simulink model "Table_airbus_v2"  (R2021b)
settings: Solver=VariableStepAuto  StartTime=0.0  StopTime=60*1.5  MaxStep=0.1  RelTol=0.01
undefined symbols (not defined in the file): X, Y, Z
libraries: sm_lib x907, fl_lib x68, nesl_utility x53, sdl_lib x10, simulink x7, ee_lib x7, slpidlib x6, simulink_extras x4
(part 4 of 18)

== system Table_airbus_v2/Vérin électrique Levage/Capteur mecanique Z1 ==
  Bus Creator : BusCreator  Inputs=4
  Ideal Rotational Motion Sensor1 : fl_lib/Mechanical/Mechanical Sensors/Ideal Rotational Motion Sensor  wrap_angle=simscape.enum.onoff.off  offset=0 deg
  Ideal Torque Sensor1 : fl_lib/Mechanical/Mechanical Sensors/Ideal Torque Sensor
  Mechanical Rotational Reference6 : fl_lib/Mechanical/Rotational Elements/Mechanical Rotational Reference
  PS Terminator : fl_lib/Physical Signals/Sinks/PS Terminator
  PS-Simulink1 : nesl_utility/PS-Simulink Converter  PhysicalDomain=network_engine_domain  SubClassName=ps_output  LeftPortType=input  RightPortType=output  PseudoPeriodic=off  Frequencies=[]  Unit=rad/s  AffineConversion=off
      settings: SourceProductBaseCode=PW,SS
  PS-Simulink4 : nesl_utility/PS-Simulink Converter  PhysicalDomain=network_engine_domain  SubClassName=ps_output  LeftPortType=input  RightPortType=output  PseudoPeriodic=off  Frequencies=[]  Unit=N*m  AffineConversion=off
      settings: SourceProductBaseCode=PW,SS
  PS-Simulink5 : nesl_utility/PS-Simulink Converter  PhysicalDomain=network_engine_domain  SubClassName=ps_output  LeftPortType=input  RightPortType=output  PseudoPeriodic=off  Frequencies=[]  Unit=rpm  AffineConversion=off
      settings: SourceProductBaseCode=PW,SS
  Product : Product
  Sortie : PMIOPort  Side=Right
  Entree : PMIOPort  Port=2  Side=Left
  Bus : Outport  VectorParamsAs1DForOutWhenUnconnected=off
  wires:
  Product/1 -> Bus Creator/4  "puissance en W"
  Bus Creator/1 -> Bus/1
  PS-Simulink4/1 -> Bus Creator/1, Product/2  "Couple Nm"
  PS-Simulink1/1 -> Bus Creator/2, Product/1  "vitesse en rad/s"
  PS-Simulink5/1 -> Bus Creator/3  "vitesse en tr/mn"
  connections:
  PS Terminator/LConn1 -- Ideal Rotational Motion Sensor1/RConn3
  Sortie/RConn1 -- Ideal Torque Sensor1/RConn1
  Mechanical Rotational Reference6/LConn1 -- Ideal Rotational Motion Sensor1/RConn1
  Ideal Torque Sensor1/RConn2 -- PS-Simulink4/LConn1
  Entree/RConn1 -- Ideal Rotational Motion Sensor1/LConn1 -- Ideal Torque Sensor1/LConn1
  Ideal Rotational Motion Sensor1/RConn2 -- PS-Simulink1/LConn1 -- PS-Simulink5/LConn1

== system Table_airbus_v2/Vérin électrique Levage/Capteur mecanique Z2 ==
  Bus Creator : BusCreator  Inputs=4
  Ideal Rotational Motion Sensor1 : fl_lib/Mechanical/Mechanical Sensors/Ideal Rotational Motion Sensor  wrap_angle=simscape.enum.onoff.off  offset=0 deg
  Ideal Torque Sensor1 : fl_lib/Mechanical/Mechanical Sensors/Ideal Torque Sensor
  Mechanical Rotational Reference6 : fl_lib/Mechanical/Rotational Elements/Mechanical Rotational Reference
  PS Terminator : fl_lib/Physical Signals/Sinks/PS Terminator
  PS-Simulink1 : nesl_utility/PS-Simulink Converter  PhysicalDomain=network_engine_domain  SubClassName=ps_output  LeftPortType=input  RightPortType=output  PseudoPeriodic=off  Frequencies=[]  Unit=rad/s  AffineConversion=off
      settings: SourceProductBaseCode=PW,SS
  PS-Simulink4 : nesl_utility/PS-Simulink Converter  PhysicalDomain=network_engine_domain  SubClassName=ps_output  LeftPortType=input  RightPortType=output  PseudoPeriodic=off  Frequencies=[]  Unit=N*m  AffineConversion=off
      settings: SourceProductBaseCode=PW,SS
  PS-Simulink5 : nesl_utility/PS-Simulink Converter  PhysicalDomain=network_engine_domain  SubClassName=ps_output  LeftPortType=input  RightPortType=output  PseudoPeriodic=off  Frequencies=[]  Unit=rpm  AffineConversion=off
      settings: SourceProductBaseCode=PW,SS
  Product : Product
  Sortie : PMIOPort  Side=Right
  Entree : PMIOPort  Port=2  Side=Left
  Bus : Outport  VectorParamsAs1DForOutWhenUnconnected=off
  wires:
  PS-Simulink5/1 -> Bus Creator/3  "vitesse en tr/mn"
  PS-Simulink1/1 -> Product/1, Bus Creator/2  "vitesse en rad/s"
  PS-Simulink4/1 -> Product/2, Bus Creator/1  "Couple Nm"
  Bus Creator/1 -> Bus/1
  Product/1 -> Bus Creator/4  "puissance en W"
  connections:
  PS-Simulink5/LConn1 -- PS-Simulink1/LConn1 -- Ideal Rotational Motion Sensor1/RConn2
  Ideal Torque Sensor1/LConn1 -- Ideal Rotational Motion Sensor1/LConn1 -- Entree/RConn1
  Ideal Torque Sensor1/RConn2 -- PS-Simulink4/LConn1
  Mechanical Rotational Reference6/LConn1 -- Ideal Rotational Motion Sensor1/RConn1
  Sortie/RConn1 -- Ideal Torque Sensor1/RConn1
  PS Terminator/LConn1 -- Ideal Rotational Motion Sensor1/RConn3

== system Table_airbus_v2/Vérin électrique Levage/Capteur mecanique Z3 ==
  Bus Creator : BusCreator  Inputs=4
  Ideal Rotational Motion Sensor1 : fl_lib/Mechanical/Mechanical Sensors/Ideal Rotational Motion Sensor  wrap_angle=simscape.enum.onoff.off  offset=0 deg
  Ideal Torque Sensor1 : fl_lib/Mechanical/Mechanical Sensors/Ideal Torque Sensor
  Mechanical Rotational Reference6 : fl_lib/Mechanical/Rotational Elements/Mechanical Rotational Reference
  PS Terminator : fl_lib/Physical Signals/Sinks/PS Terminator
  PS-Simulink1 : nesl_utility/PS-Simulink Converter  PhysicalDomain=network_engine_domain  SubClassName=ps_output  LeftPortType=input  RightPortType=output  PseudoPeriodic=off  Frequencies=[]  Unit=rad/s  AffineConversion=off
      settings: SourceProductBaseCode=PW,SS
  PS-Simulink4 : nesl_utility/PS-Simulink Converter  PhysicalDomain=network_engine_domain  SubClassName=ps_output  LeftPortType=input  RightPortType=output  PseudoPeriodic=off  Frequencies=[]  Unit=N*m  AffineConversion=off
      settings: SourceProductBaseCode=PW,SS
  PS-Simulink5 : nesl_utility/PS-Simulink Converter  PhysicalDomain=network_engine_domain  SubClassName=ps_output  LeftPortType=input  RightPortType=output  PseudoPeriodic=off  Frequencies=[]  Unit=rpm  AffineConversion=off
      settings: SourceProductBaseCode=PW,SS
  Product : Product
  Sortie : PMIOPort  Side=Right
  Entree : PMIOPort  Port=2  Side=Left
  Bus : Outport  VectorParamsAs1DForOutWhenUnconnected=off
  wires:
  Product/1 -> Bus Creator/4  "puissance en W"
  Bus Creator/1 -> Bus/1
  PS-Simulink4/1 -> Bus Creator/1, Product/2  "Couple Nm"
  PS-Simulink1/1 -> Bus Creator/2, Product/1  "vitesse en rad/s"
  PS-Simulink5/1 -> Bus Creator/3  "vitesse en tr/mn"
  connections:
  PS Terminator/LConn1 -- Ideal Rotational Motion Sensor1/RConn3
  Sortie/RConn1 -- Ideal Torque Sensor1/RConn1
  Mechanical Rotational Reference6/LConn1 -- Ideal Rotational Motion Sensor1/RConn1
  Ideal Torque Sensor1/RConn2 -- PS-Simulink4/LConn1
  Entree/RConn1 -- Ideal Rotational Motion Sensor1/LConn1 -- Ideal Torque Sensor1/LConn1
  Ideal Rotational Motion Sensor1/RConn2 -- PS-Simulink1/LConn1 -- PS-Simulink5/LConn1

== system Table_airbus_v2/Vérin électrique Levage/Capteur mecanique Z4 ==
  Bus Creator : BusCreator  Inputs=3
  Ideal Force Sensor : fl_lib/Mechanical/Mechanical Sensors/Ideal Force Sensor
  Ideal Translational Motion Sensor : fl_lib/Mechanical/Mechanical Sensors/Ideal Translational Motion Sensor  offset=0 m
  Mechanical Translational Reference : fl_lib/Mechanical/Translational Elements/Mechanical Translational Reference
  PS-Simulink1 : nesl_utility/PS-Simulink Converter  PhysicalDomain=network_engine_domain  SubClassName=ps_output  LeftPortType=input  RightPortType=output  PseudoPeriodic=off  Frequencies=[]  Unit=m/s  AffineConversion=off
      settings: SourceProductBaseCode=PW,SS
  PS-Simulink4 : nesl_utility/PS-Simulink Converter  PhysicalDomain=network_engine_domain  SubClassName=ps_output  LeftPortType=input  RightPortType=output  PseudoPeriodic=off  Frequencies=[]  Unit=N  AffineConversion=off
      settings: SourceProductBaseCode=PW,SS
  Product : Product
  Sortie : PMIOPort  Side=Right
  Entree : PMIOPort  Port=2  Side=Left
  Position tige : PMIOPort  Port=3  Side=Right
  Bus : Outport  VectorParamsAs1DForOutWhenUnconnected=off
  wires:
  PS-Simulink1/1 -> Product/1, Bus Creator/2  "vitesse en m/s"
  PS-Simulink4/1 -> Product/2, Bus Creator/1  "Force en N"
  Bus Creator/1 -> Bus/1
  Product/1 -> Bus Creator/3  "puissance en W"
  connections:
  PS-Simulink1/LConn1 -- Ideal Translational Motion Sensor/RConn2
  Entree/RConn1 -- Ideal Translational Motion Sensor/LConn1 -- Ideal Force Sensor/LConn1
  PS-Simulink4/LConn1 -- Ideal Force Sensor/RConn2
  Mechanical Translational Reference/LConn1 -- Ideal Translational Motion Sensor/RConn1
  Position tige/RConn1 -- Ideal Translational Motion Sensor/RConn3
  Ideal Force Sensor/RConn1 -- Sortie/RConn1

== system Table_airbus_v2/Vérin électrique Levage/Frein levage ==
  freinage : Inport
  Constant1 : Constant  Value=240
  Constant2 : Constant  Value=0
  Loaded-Contact Rotational Friction : sdl_lib/Brakes & Detents/Rotational/Loaded-Contact Rotational Friction  geometry_model=1  r_eff=50 mm  d_o=150 mm  d_i=100 mm  friction_model=1  mu_w_vector=[ 0 0.1 0.2 0.3 0.4 0.5 1 2 5 10 100 1000 ] rad/s  temperature_TLU=[280, 300, 320] K  mu_static=0.21  mu_static_vector=[.4, .38, .36]  mu_coulomb=0.2  mu_coulomb_vector=[ 0.29 0.28 0.26 0.22 0.21 0.2 0.2 0.19 0.19 0.19 0.19 0.19 ]  mu_coulomb_temp_vector=[.3, .28, .25]  mu_coulomb_matrix=[.34, .32, .3; .3, .28, .25; .25, .2, .15]  mu_interp_method=1  mu_extrap_method=1  w_tol=0.001 rad/s  force_min=0.01 N  mu_visc=0 N*m/(rad/s)  initial_state_locked=0  enable_faults=simscape.enum.onoff.off  fault_type=sdl.enum.clutchFault.lock  external_fault=simscape.enum.onoff.off  temporal_fault=simscape.enum.onoff.off  fault_time=5 s  report_fault=simscape.enum.assert.action.none  thermal_mass=50 kJ/K  T_init=300 K
      settings: SourceProductBaseCode=LD  InternalSimscapePortConfiguration="{\"Bottom\":[],\"Left\":[{\"id\":\"N\",\"label\":\"N\",\"type\":\"input\"},{\"id\":\"B\",\"label\":\"B\",\"type\":\"foundation.mechanical.rotational.rotational\"}],\"Right\":[{\"id\":\"F\",\"label\":\"F\",\"type\":\"foundation.mechanical.rotational.rotational\"}],\"Top\":[]}"
  Mechanical Rotational Reference2 : fl_lib/Mechanical/Rotational Elements/Mechanical Rotational Reference
  Simulink-PS Converter : nesl_utility/Simulink-PS Converter  PhysicalDomain=network_engine_domain  SubClassName=ps_input  LeftPortType=input  RightPortType=output  PseudoPeriodic=off  Frequencies=[]  NoiseDistribution=none  NoiseParameters=[]  Unit=N  AffineConversion=off  FilteringAndDerivatives=filter  SimscapeFilterOrder=1  InputFilterTimeConstant=0.001  UdotUserProvided=1
      settings: SourceProductBaseCode=PW,SS
  Switch1 : Switch  Criteria=u2 > Threshold  Threshold=0.5
  Torsional Spring-Damper : sdl_lib/Couplings & Drives/Torsional Spring-Damper  k=1000 N*m/rad  mu_visc=10 N*m/(rad/s)  trq_coulomb=0 N*m  static_kinetic_ratio=1.1  w_tol=0.001 rad/s  model_hardstop=0  upper_bound=10 deg  lower_bound=-10 deg  k_endstop=1e6 N*m/rad  D_endstop=10 N*m/(rad/s)  hardstop_model=1  transition=0.001 rad  x0=0 deg
      settings: SourceProductBaseCode=LD  InternalSimscapePortConfiguration="{\"Bottom\":[],\"Left\":[{\"id\":\"R\",\"label\":\"R\",\"type\":\"foundation.mechanical.rotational.rotational\"}],\"Right\":[{\"id\":\"C\",\"label\":\"C\",\"type\":\"foundation.mechanical.rotational.rotational\"}],\"Top\":[]}"
  rotor : PMIOPort  Side=Right
  wires:
  Constant2/1 -> Switch1/3
  Constant1/1 -> Switch1/1
  Switch1/1 -> Simulink-PS Converter/1
  freinage/1 -> Switch1/2
  connections:
  Loaded-Contact Rotational Friction/RConn1 -- Torsional Spring-Damper/LConn1
  Loaded-Contact Rotational Friction/LConn2 -- Mechanical Rotational Reference2/LConn1
  Loaded-Contact Rotational Friction/LConn1 -- Simulink-PS Converter/RConn1
  Torsional Spring-Damper/RConn1 -- rotor/RConn1

== system Table_airbus_v2/Hacheur 4 Quadrants Unipolaire moyen Inc/Hacheur 4 Q/Capteur électrique hacheur ==
  Bus Creator : BusCreator  Inputs=3
  Current Sensor1 : fl_lib/Electrical/Electrical Sensors/Current Sensor
  PS-Simulink1 : nesl_utility/PS-Simulink Converter  PhysicalDomain=network_engine_domain  SubClassName=ps_output  LeftPortType=input  RightPortType=output  PseudoPeriodic=off  Frequencies=[]  Unit=V  AffineConversion=off
      settings: SourceProductBaseCode=PW,SS
  PS-Simulink4 : nesl_utility/PS-Simulink Converter  PhysicalDomain=network_engine_domain  SubClassName=ps_output  LeftPortType=input  RightPortType=output  PseudoPeriodic=off  Frequencies=[]  Unit=A  AffineConversion=off
      settings: SourceProductBaseCode=PW,SS
  Product : Product
  Voltage Sensor : fl_lib/Electrical/Electrical Sensors/Voltage Sensor
  S+ : PMIOPort  Side=Right
  E+ : PMIOPort  Port=2  Side=Left
  E- : PMIOPort  Port=3  Side=Left
  Bus : Outport  VectorParamsAs1DForOutWhenUnconnected=off
  wires:
  Product/1 -> Bus Creator/3  "puissance en W"
  Bus Creator/1 -> Bus/1
  PS-Simulink4/1 -> Product/1, Bus Creator/1  "Intensité A"
  PS-Simulink1/1 -> Product/2, Bus Creator/2  "tension en V"
  connections:
  PS-Simulink1/LConn1 -- Voltage Sensor/RConn1
  PS-Simulink4/LConn1 -- Current Sensor1/RConn1
  E+/RConn1 -- Current Sensor1/LConn1
  S+/RConn1 -- Current Sensor1/RConn2 -- Voltage Sensor/LConn1
  E-/RConn1 -- Voltage Sensor/RConn2

== system Table_airbus_v2/Hacheur 4 Quadrants Unipolaire moyen lev/Hacheur 4 Q/Capteur électrique hacheur ==
  Bus Creator : BusCreator  Inputs=3
  Current Sensor1 : fl_lib/Electrical/Electrical Sensors/Current Sensor
  PS-Simulink1 : nesl_utility/PS-Simulink Converter  PhysicalDomain=network_engine_domain  SubClassName=ps_output  LeftPortType=input  RightPortType=output  PseudoPeriodic=off  Frequencies=[]  Unit=V  AffineConversion=off
      settings: SourceProductBaseCode=PW,SS
  PS-Simulink4 : nesl_utility/PS-Simulink Converter  PhysicalDomain=network_engine_domain  SubClassName=ps_output  LeftPortType=input  RightPortType=output  PseudoPeriodic=off  Frequencies=[]  Unit=A  AffineConversion=off
      settings: SourceProductBaseCode=PW,SS
  Product : Product
  Voltage Sensor : fl_lib/Electrical/Electrical Sensors/Voltage Sensor
  S+ : PMIOPort  Side=Right
  E+ : PMIOPort  Port=2  Side=Left
  E- : PMIOPort  Port=3  Side=Left
  Bus : Outport  VectorParamsAs1DForOutWhenUnconnected=off
  wires:
  PS-Simulink1/1 -> Bus Creator/2, Product/2  "tension en V"
  PS-Simulink4/1 -> Bus Creator/1, Product/1  "Intensité A"
  Bus Creator/1 -> Bus/1
  Product/1 -> Bus Creator/3  "puissance en W"
  connections:
  E-/RConn1 -- Voltage Sensor/RConn2
  Voltage Sensor/LConn1 -- Current Sensor1/RConn2 -- S+/RConn1
  E+/RConn1 -- Current Sensor1/LConn1
  PS-Simulink4/LConn1 -- Current Sensor1/RConn1
  PS-Simulink1/LConn1 -- Voltage Sensor/RConn1

== system Table_airbus_v2/Modèle mécanique1/Table/Corps_v_rin_inclinaison_1_RIGID ==
  ReferenceFrame : sm_lib/Frames and Transforms/Reference Frame
  Transform : sm_lib/Frames and Transforms/Rigid Transform  TranslationMethod=Cartesian  TranslationStandardOffset=0  TranslationLengthUnit=mm  TranslationStandardAxis=+Z  TranslationCartesianOffset=[581.58897838011512 -79.972299999999905 18.779086684198781]  TranslationROffset=0  TranslationROffsetUnits=m  TranslationZOffset=0  TranslationZOffsetUnits=m  TranslationThetaOffset=0  TranslationThetaOffsetUnits=deg  RotationMethod=ArbitraryAxis  RotationAngleUnits=rad  RotationStandardAxis=+Z  RotationAngle=2.0943951023931957  RotationArbitraryAxis=[0.57735026918962573 0.57735026918962584 0.57735026918962573]  FollAlignAxisA=+X  BaseAlignAxisA=+Y  FollAlignAxisB=+Y  BaseAlignAxisB=+Z  RotationSequenceAxes=FollowerAxes  RotationSequence=XYX  RotationSequenceAngles=[0 0 0]  RotationSequenceAnglesUnits=deg  RotationMatrix=[1 0 0; 0 1 0; 0 0 1]
  Transform1 : sm_lib/Frames and Transforms/Rigid Transform  TranslationMethod=Cartesian  TranslationStandardOffset=0  TranslationLengthUnit=mm  TranslationStandardAxis=+Z  TranslationCartesianOffset=[16.943688345754151 -124.27970000002227 18.779161135203918]  TranslationROffset=0  TranslationROffsetUnits=m  TranslationZOffset=0  TranslationZOffsetUnits=m  TranslationThetaOffset=0  TranslationThetaOffsetUnits=deg  RotationMethod=ArbitraryAxis  RotationAngleUnits=rad  RotationStandardAxis=+Z  RotationAngle=2.0943951023931957  RotationArbitraryAxis=[0.57735026918962584 -0.57735026918962551 0.57735026918962595]  FollAlignAxisA=+X  BaseAlignAxisA=+Y  FollAlignAxisB=+Y  BaseAlignAxisB=+Z  RotationSequenceAxes=FollowerAxes  RotationSequence=XYX  RotationSequenceAngles=[0 0 0]  RotationSequenceAnglesUnits=deg  RotationMatrix=[1 0 0; 0 1 0; 0 0 1]
  Transform2 : sm_lib/Frames and Transforms/Rigid Transform  TranslationMethod=Cartesian  TranslationStandardOffset=0  TranslationLengthUnit=mm  TranslationStandardAxis=+Z  TranslationCartesianOffset=[223.357 -79.97229999999999 92.199100000000001]  TranslationROffset=0  TranslationROffsetUnits=m  TranslationZOffset=0  TranslationZOffsetUnits=m  TranslationThetaOffset=0  TranslationThetaOffsetUnits=deg  RotationMethod=ArbitraryAxis  RotationAngleUnits=rad  RotationStandardAxis=+Z  RotationAngle=3.1415926535897931  RotationArbitraryAxis=[-0.70710678118654746 -5.2401915786782071e-17 -0.70710678118654757]  FollAlignAxisA=+X  BaseAlignAxisA=+Y  FollAlignAxisB=+Y  BaseAlignAxisB=+Z  RotationSequenceAxes=FollowerAxes  RotationSequence=XYX  RotationSequenceAngles=[0 0 0]  RotationSequenceAnglesUnits=deg  RotationMatrix=[1 0 0; 0 1 0; 0 0 1]
  Transform3 : sm_lib/Frames and Transforms/Rigid Transform  TranslationMethod=Cartesian  TranslationStandardOffset=0  TranslationLengthUnit=mm  TranslationStandardAxis=+Z  TranslationCartesianOffset=[61.256599999999999 -79.97229999999999 18.7791]  TranslationROffset=0  TranslationROffsetUnits=m  TranslationZOffset=0  TranslationZOffsetUnits=m  TranslationThetaOffset=0  TranslationThetaOffsetUnits=deg  RotationMethod=ArbitraryAxis  RotationAngleUnits=rad  RotationStandardAxis=+Z  RotationAngle=1.6178481128137681  RotationArbitraryAxis=[0.21194708467810194 -0.21194708467810194 0.95402141830930975]  FollAlignAxisA=+X  BaseAlignAxisA=+Y  FollAlignAxisB=+Y  BaseAlignAxisB=+Z  RotationSequenceAxes=FollowerAxes  RotationSequence=XYX  RotationSequenceAngles=[0 0 0]  RotationSequenceAnglesUnits=deg  RotationMatrix=[1 0 0; 0 1 0; 0 0 1]
  Transform4 : sm_lib/Frames and Transforms/Rigid Transform  TranslationMethod=Cartesian  TranslationStandardOffset=0  TranslationLengthUnit=mm  TranslationStandardAxis=+Z  TranslationCartesianOffset=[16.944099999999999 -79.97229999999999 18.7791]  TranslationROffset=0  TranslationROffsetUnits=m  TranslationZOffset=0  TranslationZOffsetUnits=m  TranslationThetaOffset=0  TranslationThetaOffsetUnits=deg  RotationMethod=None  RotationAngleUnits=deg  RotationStandardAxis=+Z  RotationAngle=0  RotationArbitraryAxis=[0 0 1]  FollAlignAxisA=+X  BaseAlignAxisA=+Y  FollAlignAxisB=+Y  BaseAlignAxisB=+Z  RotationSequenceAxes=FollowerAxes  RotationSequence=XYX  RotationSequenceAngles=[0 0 0]  RotationSequenceAnglesUnits=deg  RotationMatrix=[1 0 0; 0 1 0; 0 0 1]
  Transform5 : sm_lib/Frames and Transforms/Rigid Transform  TranslationMethod=Cartesian  TranslationStandardOffset=0  TranslationLengthUnit=mm  TranslationStandardAxis=+Z  TranslationCartesianOffset=[117.25700000000001 -79.97229999999999 18.7791]  TranslationROffset=0  TranslationROffsetUnits=m  TranslationZOffset=0  TranslationZOffsetUnits=m  TranslationThetaOffset=0  TranslationThetaOffsetUnits=deg  RotationMethod=ArbitraryAxis  RotationAngleUnits=rad  RotationStandardAxis=+Z  RotationAngle=3.1415926535897931  RotationArbitraryAxis=[0 0.97311979050629582 0.2302995295804641]  FollAlignAxisA=+X  BaseAlignAxisA=+Y  FollAlignAxisB=+Y  BaseAlignAxisB=+Z  RotationSequenceAxes=FollowerAxes  RotationSequence=XYX  RotationSequenceAngles=[0 0 0]  RotationSequenceAnglesUnits=deg  RotationMatrix=[1 0 0; 0 1 0; 0 0 1]
  x15060_Ecrou_24_Ecrou_Hm_M16_1_RIGID : Subsystem
  x15060_M_01073_Interface_ar_verin_AA_DEFAULT_1_RIGID : Subsystem
  x15060_NLM_Embout_a_rotule_M16_Pas_a_droite_27627_16_1_RIGID : Subsystem
  x15060_Verin_LA36_Course_100_mm_1_RIGID : Subsystem
  F1 : PMIOPort  Side=Left
  F : PMIOPort  Port=2  Side=Right
  connections:
  Transform5/RConn1 -- x15060_M_01073_Interface_ar_verin_AA_DEFAULT_1_RIGID/LConn1
  Transform4/RConn1 -- x15060_NLM_Embout_a_rotule_M16_Pas_a_droite_27627_16_1_RIGID/LConn1
  Transform3/RConn1 -- x15060_Ecrou_24_Ecrou_Hm_M16_1_RIGID/LConn1
  Transform2/RConn1 -- x15060_Verin_LA36_Course_100_mm_1_RIGID/LConn1
  Transform1/RConn1 -- F1/RConn1
  Transform/RConn1 -- F/RConn1
  Transform2/LConn1 -- Transform3/LConn1 -- Transform5/LConn1 -- Transform4/LConn1 -- ReferenceFrame/RConn1 -- Transform1/LConn1 -- Transform/LConn1

== system Table_airbus_v2/Modèle mécanique1/Table/Corps_v_rin_levage_1_RIGID ==
  ReferenceFrame : sm_lib/Frames and Transforms/Reference Frame
  Transform : sm_lib/Frames and Transforms/Rigid Transform  TranslationMethod=Cartesian  TranslationStandardOffset=0  TranslationLengthUnit=mm  TranslationStandardAxis=+Z  TranslationCartesianOffset=[16.948520761169686 32.492699999977624 18.777580013894262]  TranslationROffset=0  TranslationROffsetUnits=m  TranslationZOffset=0  TranslationZOffsetUnits=m  TranslationThetaOffset=0  TranslationThetaOffsetUnits=deg  RotationMethod=ArbitraryAxis  RotationAngleUnits=rad  RotationStandardAxis=+Z  RotationAngle=2.0943951023931935  RotationArbitraryAxis=[-0.57735026918962506 -0.57735026918962595 -0.5773502691896264]  FollAlignAxisA=+X  BaseAlignAxisA=+Y  FollAlignAxisB=+Y  BaseAlignAxisB=+Z  RotationSequenceAxes=FollowerAxes  RotationSequence=XYX  RotationSequenceAngles=[0 0 0]  RotationSequenceAnglesUnits=deg  RotationMatrix=[1 0 0; 0 1 0; 0 0 1]
  Transform1 : sm_lib/Frames and Transforms/Rigid Transform  TranslationMethod=Cartesian  TranslationStandardOffset=0  TranslationLengthUnit=mm  TranslationStandardAxis=+Z  TranslationCartesianOffset=[449.09427593857532 -79.972300000000033 18.776101630550443]  TranslationROffset=0  TranslationROffsetUnits=m  TranslationZOffset=0  TranslationZOffsetUnits=m  TranslationThetaOffset=0  TranslationThetaOffsetUnits=deg  RotationMethod=ArbitraryAxis  RotationAngleUnits=rad  RotationStandardAxis=+Z  RotationAngle=2.0943951023931953  RotationArbitraryAxis=[0.57735026918962551 0.57735026918962562 0.57735026918962606]  FollAlignAxisA=+X  BaseAlignAxisA=+Y  FollAlignAxisB=+Y  BaseAlignAxisB=+Z  RotationSequenceAxes=FollowerAxes  RotationSequence=XYX  RotationSequenceAngles=[0 0 0]  RotationSequenceAnglesUnits=deg  RotationMatrix=[1 0 0; 0 1 0; 0 0 1]
  Transform2 : sm_lib/Frames and Transforms/Rigid Transform  TranslationMethod=Cartesian  TranslationStandardOffset=0  TranslationLengthUnit=mm  TranslationStandardAxis=+Z  TranslationCartesianOffset=[55.8872 -79.97229999999999 18.7791]  TranslationROffset=0  TranslationROffsetUnits=m  TranslationZOffset=0  TranslationZOffsetUnits=m  TranslationThetaOffset=0  TranslationThetaOffsetUnits=deg  RotationMethod=ArbitraryAxis  RotationAngleUnits=rad  RotationStandardAxis=+Z  RotationAngle=1.6178481128137681  RotationArbitraryAxis=[0.21194708467810197 -0.21194708467810194 0.95402141830930975]  FollAlignAxisA=+X  BaseAlignAxisA=+Y  FollAlignAxisB=+Y  BaseAlignAxisB=+Z  RotationSequenceAxes=FollowerAxes  RotationSequence=XYX  RotationSequenceAngles=[0 0 0]  RotationSequenceAnglesUnits=deg  RotationMatrix=[1 0 0; 0 1 0; 0 0 1]
  Transform3 : sm_lib/Frames and Transforms/Rigid Transform  TranslationMethod=Cartesian  TranslationStandardOffset=0  TranslationLengthUnit=mm  TranslationStandardAxis=+Z  TranslationCartesianOffset=[111.887 -79.97229999999999 18.7791]  TranslationROffset=0  TranslationROffsetUnits=m  TranslationZOffset=0  TranslationZOffsetUnits=m  TranslationThetaOffset=0  TranslationThetaOffsetUnits=deg  RotationMethod=ArbitraryAxis  RotationAngleUnits=rad  RotationStandardAxis=+Z  RotationAngle=3.1415926535897931  RotationArbitraryAxis=[0 0.36955459314218925 0.92920901991291016]  FollAlignAxisA=+X  BaseAlignAxisA=+Y  FollAlignAxisB=+Y  BaseAlignAxisB=+Z  RotationSequenceAxes=FollowerAxes  RotationSequence=XYX  RotationSequenceAngles=[0 0 0]  RotationSequenceAnglesUnits=deg  RotationMatrix=[1 0 0; 0 1 0; 0 0 1]
  Transform4 : sm_lib/Frames and Transforms/Rigid Transform  TranslationMethod=Cartesian  TranslationStandardOffset=0  TranslationLengthUnit=mm  TranslationStandardAxis=+Z  TranslationCartesianOffset=[217.98699999999999 -6.5523399999999992 18.7791]  TranslationROffset=0  TranslationROffsetUnits=m  TranslationZOffset=0  TranslationZOffsetUnits=m  TranslationThetaOffset=0  TranslationThetaOffsetUnits=deg  RotationMethod=ArbitraryAxis  RotationAngleUnits=rad  RotationStandardAxis=+Z  RotationAngle=2.0943951023931953  RotationArbitraryAxis=[0.57735026918962584 0.57735026918962584 0.57735026918962584]  FollAlignAxisA=+X  BaseAlignAxisA=+Y  FollAlignAxisB=+Y  BaseAlignAxisB=+Z  RotationSequenceAxes=FollowerAxes  RotationSequence=XYX  RotationSequenceAngles=[0 0 0]  RotationSequenceAnglesUnits=deg  RotationMatrix=[1 0 0; 0 1 0; 0 0 1]
  Transform5 : sm_lib/Frames and Transforms/Rigid Transform  TranslationMethod=Cartesian  TranslationStandardOffset=0  TranslationLengthUnit=mm  TranslationStandardAxis=+Z  TranslationCartesianOffset=[16.944099999999999 -79.97229999999999 18.7791]  TranslationROffset=0  TranslationROffsetUnits=m  TranslationZOffset=0  TranslationZOffsetUnits=m  TranslationThetaOffset=0  TranslationThetaOffsetUnits=deg  RotationMethod=None  RotationAngleUnits=deg  RotationStandardAxis=+Z  RotationAngle=0  RotationArbitraryAxis=[0 0 1]  FollAlignAxisA=+X  BaseAlignAxisA=+Y  FollAlignAxisB=+Y  BaseAlignAxisB=+Z  RotationSequenceAxes=FollowerAxes  RotationSequence=XYX  RotationSequenceAngles=[0 0 0]  RotationSequenceAnglesUnits=deg  RotationMatrix=[1 0 0; 0 1 0; 0 0 1]
  x15060_Ecrou_24_Ecrou_Hm_M16_1_RIGID : Subsystem
  x15060_M_01073_Interface_ar_verin_AA_DEFAULT_1_RIGID : Subsystem
  x15060_NLM_Embout_a_rotule_M16_Pas_a_droite_27627_16_1_RIGID : Subsystem
  x15060_Verin_LA36_Course_100_mm_1_RIGID : Subsystem
  F : PMIOPort  Side=Left
  F1 : PMIOPort  Port=2  Side=Left
  connections:
  Transform5/RConn1 -- x15060_NLM_Embout_a_rotule_M16_Pas_a_droite_27627_16_1_RIGID/LConn1
  Transform4/RConn1 -- x15060_Verin_LA36_Course_100_mm_1_RIGID/LConn1
  Transform3/RConn1 -- x15060_M_01073_Interface_ar_verin_AA_DEFAULT_1_RIGID/LConn1
  Transform2/RConn1 -- x15060_Ecrou_24_Ecrou_Hm_M16_1_RIGID/LConn1
  Transform1/RConn1 -- F1/RConn1
  Transform/RConn1 -- F/RConn1
  Transform2/LConn1 -- Transform3/LConn1 -- Transform5/LConn1 -- Transform4/LConn1 -- ReferenceFrame/RConn1 -- Transform1/LConn1 -- Transform/LConn1

== system Table_airbus_v2/Modèle mécanique1/Table/Tige_v_rin_inclinaison_1_RIGID ==
  ReferenceFrame : sm_lib/Frames and Transforms/Reference Frame
  Transform : sm_lib/Frames and Transforms/Rigid Transform  TranslationMethod=Cartesian  TranslationStandardOffset=0  TranslationLengthUnit=mm  TranslationStandardAxis=+Z  TranslationCartesianOffset=[498.38299999999998 -79.97229999999999 18.7791]  TranslationROffset=0  TranslationROffsetUnits=m  TranslationZOffset=0  TranslationZOffsetUnits=m  TranslationThetaOffset=0  TranslationThetaOffsetUnits=deg  RotationMethod=ArbitraryAxis  RotationAngleUnits=deg  RotationStandardAxis=+Z  RotationAngle=-90  RotationArbitraryAxis=[1 0 0]  FollAlignAxisA=+X  BaseAlignAxisA=+Y  FollAlignAxisB=+Y  BaseAlignAxisB=+Z  RotationSequenceAxes=FollowerAxes  RotationSequence=XYX  RotationSequenceAngles=[0 0 0]  RotationSequenceAnglesUnits=deg  RotationMatrix=[1 0 0; 0 1 0; 0 0 1]
  Transform1 : sm_lib/Frames and Transforms/Rigid Transform  TranslationMethod=Cartesian  TranslationStandardOffset=0  TranslationLengthUnit=mm  TranslationStandardAxis=+Z  TranslationCartesianOffset=[483.03179999999998 -79.97229999999999 18.7791]  TranslationROffset=0  TranslationROffsetUnits=m  TranslationZOffset=0  TranslationZOffsetUnits=m  TranslationThetaOffset=0  TranslationThetaOffsetUnits=deg  RotationMethod=ArbitraryAxis  RotationAngleUnits=rad  RotationStandardAxis=+Z  RotationAngle=2.0943951023931953  RotationArbitraryAxis=[0.57735026918962584 0.57735026918962584 0.57735026918962584]  FollAlignAxisA=+X  BaseAlignAxisA=+Y  FollAlignAxisB=+Y  BaseAlignAxisB=+Z  RotationSequenceAxes=FollowerAxes  RotationSequence=XYX  RotationSequenceAngles=[0 0 0]  RotationSequenceAnglesUnits=deg  RotationMatrix=[1 0 0; 0 1 0; 0 0 1]
  Transform2 : sm_lib/Frames and Transforms/Rigid Transform  TranslationMethod=Cartesian  TranslationStandardOffset=0  TranslationLengthUnit=mm  TranslationStandardAxis=+Z  TranslationCartesianOffset=[468.38299999999998 -79.97229999999999 18.7791]  TranslationROffset=0  TranslationROffsetUnits=m  TranslationZOffset=0  TranslationZOffsetUnits=m  TranslationThetaOffset=0  TranslationThetaOffsetUnits=deg  RotationMethod=ArbitraryAxis  RotationAngleUnits=rad  RotationStandardAxis=+Z  RotationAngle=1.5707963267948968  RotationArbitraryAxis=[-1 -0 -0]  FollAlignAxisA=+X  BaseAlignAxisA=+Y  FollAlignAxisB=+Y  BaseAlignAxisB=+Z  RotationSequenceAxes=FollowerAxes  RotationSequence=XYX  RotationSequenceAngles=[0 0 0]  RotationSequenceAnglesUnits=deg  RotationMatrix=[1 0 0; 0 1 0; 0 0 1]
  Transform3 : sm_lib/Frames and Transforms/Rigid Transform  TranslationMethod=Cartesian  TranslationStandardOffset=0  TranslationLengthUnit=mm  TranslationStandardAxis=+Z  TranslationCartesianOffset=[468.38299999999998 -79.97229999999999 18.7791]  TranslationROffset=0  TranslationROffsetUnits=m  TranslationZOffset=0  TranslationZOffsetUnits=m  TranslationThetaOffset=0  TranslationThetaOffsetUnits=deg  RotationMethod=ArbitraryAxis  RotationAngleUnits=rad  RotationStandardAxis=+Z  RotationAngle=3.1415926535897931  RotationArbitraryAxis=[0 -0.69484755531927389 0.71915705855315692]  FollAlignAxisA=+X  BaseAlignAxisA=+Y  FollAlignAxisB=+Y  BaseAlignAxisB=+Z  RotationSequenceAxes=FollowerAxes  RotationSequence=XYX  RotationSequenceAngles=[0 0 0]  RotationSequenceAnglesUnits=deg  RotationMatrix=[1 0 0; 0 1 0; 0 0 1]
  x15060_Tige_Verin_LA36_AA_DEFAULT_1_RIGID : Subsystem
  x15060_Verin_LA36_Rotule_tige_verin_AA_DEFAULT_1_RIGID : Subsystem
  F : PMIOPort  Side=Left
  F1 : PMIOPort  Port=2  Side=Right
  connections:
  Transform3/RConn1 -- x15060_Tige_Verin_LA36_AA_DEFAULT_1_RIGID/LConn1
  Transform2/RConn1 -- x15060_Verin_LA36_Rotule_tige_verin_AA_DEFAULT_1_RIGID/LConn1
  Transform1/RConn1 -- F1/RConn1
  Transform/RConn1 -- F/RConn1
  Transform1/LConn1 -- Transform3/LConn1 -- Transform2/LConn1 -- ReferenceFrame/RConn1 -- Transform/LConn1

== system Table_airbus_v2/Modèle mécanique1/Table/Tige_v_rin_levage_1_RIGID ==
  ReferenceFrame : sm_lib/Frames and Transforms/Reference Frame
  Transform : sm_lib/Frames and Transforms/Rigid Transform  TranslationMethod=Cartesian  TranslationStandardOffset=0  TranslationLengthUnit=mm  TranslationStandardAxis=+Z  TranslationCartesianOffset=[483.03179999999998 -79.97229999999999 18.7791]  TranslationROffset=0  TranslationROffsetUnits=m  TranslationZOffset=0  TranslationZOffsetUnits=m  TranslationThetaOffset=0  TranslationThetaOffsetUnits=deg  RotationMethod=ArbitraryAxis  RotationAngleUnits=rad  RotationStandardAxis=+Z  RotationAngle=2.0943951023931953  RotationArbitraryAxis=[0.57735026918962584 0.57735026918962584 0.57735026918962584]  FollAlignAxisA=+X  BaseAlignAxisA=+Y  FollAlignAxisB=+Y  BaseAlignAxisB=+Z  RotationSequenceAxes=FollowerAxes  RotationSequence=XYX  RotationSequenceAngles=[0 0 0]  RotationSequenceAnglesUnits=deg  RotationMatrix=[1 0 0; 0 1 0; 0 0 1]
  Transform1 : sm_lib/Frames and Transforms/Rigid Transform  TranslationMethod=Cartesian  TranslationStandardOffset=0  TranslationLengthUnit=mm  TranslationStandardAxis=+Z  TranslationCartesianOffset=[498.37802463250813 -80 18.780491340163735]  TranslationROffset=0  TranslationROffsetUnits=m  TranslationZOffset=0  TranslationZOffsetUnits=m  TranslationThetaOffset=0  TranslationThetaOffsetUnits=deg  RotationMethod=ArbitraryAxis  RotationAngleUnits=rad  RotationStandardAxis=+Z  RotationAngle=1.6503241427683797  RotationArbitraryAxis=[0.92347478817432327 -0.27128796103622821 0.27128796103622921]  FollAlignAxisA=+X  BaseAlignAxisA=+Y  FollAlignAxisB=+Y  BaseAlignAxisB=+Z  RotationSequenceAxes=FollowerAxes  RotationSequence=XYX  RotationSequenceAngles=[0 0 0]  RotationSequenceAnglesUnits=deg  RotationMatrix=[1 0 0; 0 1 0; 0 0 1]
  Transform2 : sm_lib/Frames and Transforms/Rigid Transform  TranslationMethod=Cartesian  TranslationStandardOffset=0  TranslationLengthUnit=mm  TranslationStandardAxis=+Z  TranslationCartesianOffset=[468.38299999999998 -79.97229999999999 18.7791]  TranslationROffset=0  TranslationROffsetUnits=m  TranslationZOffset=0  TranslationZOffsetUnits=m  TranslationThetaOffset=0  TranslationThetaOffsetUnits=deg  RotationMethod=ArbitraryAxis  RotationAngleUnits=rad  RotationStandardAxis=+Z  RotationAngle=1.5707963267948968  RotationArbitraryAxis=[-1 -0 -0]  FollAlignAxisA=+X  BaseAlignAxisA=+Y  FollAlignAxisB=+Y  BaseAlignAxisB=+Z  RotationSequenceAxes=FollowerAxes  RotationSequence=XYX  RotationSequenceAngles=[0 0 0]  RotationSequenceAnglesUnits=deg  RotationMatrix=[1 0 0; 0 1 0; 0 0 1]
  Transform3 : sm_lib/Frames and Transforms/Rigid Transform  TranslationMethod=Cartesian  TranslationStandardOffset=0  TranslationLengthUnit=mm  TranslationStandardAxis=+Z  TranslationCartesianOffset=[468.38299999999998 -79.97229999999999 18.7791]  TranslationROffset=0  TranslationROffsetUnits=m  TranslationZOffset=0  TranslationZOffsetUnits=m  TranslationThetaOffset=0  TranslationThetaOffsetUnits=deg  RotationMethod=ArbitraryAxis  RotationAngleUnits=rad  RotationStandardAxis=+Z  RotationAngle=3.1415926535897931  RotationArbitraryAxis=[0 -0.69484755531927389 0.71915705855315692]  FollAlignAxisA=+X  BaseAlignAxisA=+Y  FollAlignAxisB=+Y  BaseAlignAxisB=+Z  RotationSequenceAxes=FollowerAxes  RotationSequence=XYX  RotationSequenceAngles=[0 0 0]  RotationSequenceAnglesUnits=deg  RotationMatrix=[1 0 0; 0 1 0; 0 0 1]
  x15060_Tige_Verin_LA36_AA_DEFAULT_1_RIGID : Subsystem
  x15060_Verin_LA36_Rotule_tige_verin_AA_DEFAULT_1_RIGID : Subsystem
  F1 : PMIOPort  Side=Left
  F : PMIOPort  Port=2  Side=Right
  connections:
  Transform3/RConn1 -- x15060_Tige_Verin_LA36_AA_DEFAULT_1_RIGID/LConn1
  Transform2/RConn1 -- x15060_Verin_LA36_Rotule_tige_verin_AA_DEFAULT_1_RIGID/LConn1
  Transform1/RConn1 -- F1/RConn1
  Transform/RConn1 -- F/RConn1
  Transform3/LConn1 -- Transform2/LConn1 -- ReferenceFrame/RConn1 -- Transform1/LConn1 -- Transform/LConn1

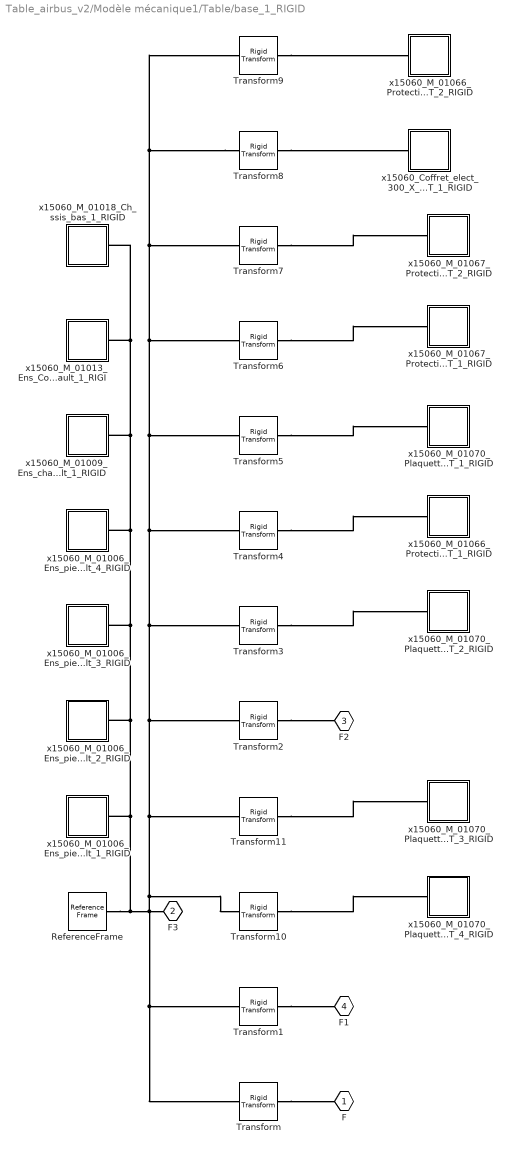
== system Table_airbus_v2/Modèle mécanique1/Table/base_1_RIGID ==
  ReferenceFrame : sm_lib/Frames and Transforms/Reference Frame
  Transform : sm_lib/Frames and Transforms/Rigid Transform  TranslationMethod=Cartesian  TranslationStandardOffset=0  TranslationLengthUnit=mm  TranslationStandardAxis=+Z  TranslationCartesianOffset=[-1242 73.964999999999918 -35]  TranslationROffset=0  TranslationROffsetUnits=m  TranslationZOffset=0  TranslationZOffsetUnits=m  TranslationThetaOffset=0  TranslationThetaOffsetUnits=deg  RotationMethod=ArbitraryAxis  RotationAngleUnits=rad  RotationStandardAxis=+Z  RotationAngle=2.0943951023931953  RotationArbitraryAxis=[-0.57735026918962562 -0.57735026918962595 -0.57735026918962562]  FollAlignAxisA=+X  BaseAlignAxisA=+Y  FollAlignAxisB=+Y  BaseAlignAxisB=+Z  RotationSequenceAxes=FollowerAxes  RotationSequence=XYX  RotationSequenceAngles=[0 0 0]  RotationSequenceAnglesUnits=deg  RotationMatrix=[1 0 0; 0 1 0; 0 0 1]
  Transform1 : sm_lib/Frames and Transforms/Rigid Transform  TranslationMethod=Cartesian  TranslationStandardOffset=0  TranslationLengthUnit=mm  TranslationStandardAxis=+Z  TranslationCartesianOffset=[-1320 -193.8074 -14.000000000000002]  TranslationROffset=0  TranslationROffsetUnits=m  TranslationZOffset=0  TranslationZOffsetUnits=m  TranslationThetaOffset=0  TranslationThetaOffsetUnits=deg  RotationMethod=ArbitraryAxis  RotationAngleUnits=rad  RotationStandardAxis=+Z  RotationAngle=2.0943951023931953  RotationArbitraryAxis=[0.57735026918962584 -0.57735026918962584 0.57735026918962584]  FollAlignAxisA=+X  BaseAlignAxisA=+Y  FollAlignAxisB=+Y  BaseAlignAxisB=+Z  RotationSequenceAxes=FollowerAxes  RotationSequence=XYX  RotationSequenceAngles=[0 0 0]  RotationSequenceAnglesUnits=deg  RotationMatrix=[1 0 0; 0 1 0; 0 0 1]
  Transform10 : sm_lib/Frames and Transforms/Rigid Transform  TranslationMethod=Cartesian  TranslationStandardOffset=0  TranslationLengthUnit=mm  TranslationStandardAxis=+Z  TranslationCartesianOffset=[-200 -325 -60]  TranslationROffset=0  TranslationROffsetUnits=m  TranslationZOffset=0  TranslationZOffsetUnits=m  TranslationThetaOffset=0  TranslationThetaOffsetUnits=deg  RotationMethod=ArbitraryAxis  RotationAngleUnits=rad  RotationStandardAxis=+Z  RotationAngle=3.1415926535897891  RotationArbitraryAxis=[0 1 0]  FollAlignAxisA=+X  BaseAlignAxisA=+Y  FollAlignAxisB=+Y  BaseAlignAxisB=+Z  RotationSequenceAxes=FollowerAxes  RotationSequence=XYX  RotationSequenceAngles=[0 0 0]  RotationSequenceAnglesUnits=deg  RotationMatrix=[1 0 0; 0 1 0; 0 0 1]
  Transform11 : sm_lib/Frames and Transforms/Rigid Transform  TranslationMethod=Cartesian  TranslationStandardOffset=0  TranslationLengthUnit=mm  TranslationStandardAxis=+Z  TranslationCartesianOffset=[-200 215 -60]  TranslationROffset=0  TranslationROffsetUnits=m  TranslationZOffset=0  TranslationZOffsetUnits=m  TranslationThetaOffset=0  TranslationThetaOffsetUnits=deg  RotationMethod=ArbitraryAxis  RotationAngleUnits=rad  RotationStandardAxis=+Z  RotationAngle=3.1415926535897891  RotationArbitraryAxis=[0 1 0]  FollAlignAxisA=+X  BaseAlignAxisA=+Y  FollAlignAxisB=+Y  BaseAlignAxisB=+Z  RotationSequenceAxes=FollowerAxes  RotationSequence=XYX  RotationSequenceAngles=[0 0 0]  RotationSequenceAnglesUnits=deg  RotationMatrix=[1 0 0; 0 1 0; 0 0 1]
  Transform2 : sm_lib/Frames and Transforms/Rigid Transform  TranslationMethod=Cartesian  TranslationStandardOffset=0  TranslationLengthUnit=mm  TranslationStandardAxis=+Z  TranslationCartesianOffset=[-1400 -138.965 121.00000000000195]  TranslationROffset=0  TranslationROffsetUnits=m  TranslationZOffset=0  TranslationZOffsetUnits=m  TranslationThetaOffset=0  TranslationThetaOffsetUnits=deg  RotationMethod=ArbitraryAxis  RotationAngleUnits=rad  RotationStandardAxis=+Z  RotationAngle=2.0943951023931953  RotationArbitraryAxis=[0.57735026918962584 -0.57735026918962584 0.57735026918962584]  FollAlignAxisA=+X  BaseAlignAxisA=+Y  FollAlignAxisB=+Y  BaseAlignAxisB=+Z  RotationSequenceAxes=FollowerAxes  RotationSequence=XYX  RotationSequenceAngles=[0 0 0]  RotationSequenceAnglesUnits=deg  RotationMatrix=[1 0 0; 0 1 0; 0 0 1]
  Transform3 : sm_lib/Frames and Transforms/Rigid Transform  TranslationMethod=Cartesian  TranslationStandardOffset=0  TranslationLengthUnit=mm  TranslationStandardAxis=+Z  TranslationCartesianOffset=[-550 -325 -60]  TranslationROffset=0  TranslationROffsetUnits=m  TranslationZOffset=0  TranslationZOffsetUnits=m  TranslationThetaOffset=0  TranslationThetaOffsetUnits=deg  RotationMethod=ArbitraryAxis  RotationAngleUnits=rad  RotationStandardAxis=+Z  RotationAngle=3.1415926535897931  RotationArbitraryAxis=[1 -6.2449999999999997e-17 0]  FollAlignAxisA=+X  BaseAlignAxisA=+Y  FollAlignAxisB=+Y  BaseAlignAxisB=+Z  RotationSequenceAxes=FollowerAxes  RotationSequence=XYX  RotationSequenceAngles=[0 0 0]  RotationSequenceAnglesUnits=deg  RotationMatrix=[1 0 0; 0 1 0; 0 0 1]
  Transform4 : sm_lib/Frames and Transforms/Rigid Transform  TranslationMethod=Cartesian  TranslationStandardOffset=0  TranslationLengthUnit=mm  TranslationStandardAxis=+Z  TranslationCartesianOffset=[-1740 -415 31]  TranslationROffset=0  TranslationROffsetUnits=m  TranslationZOffset=0  TranslationZOffsetUnits=m  TranslationThetaOffset=0  TranslationThetaOffsetUnits=deg  RotationMethod=None  RotationAngleUnits=deg  RotationStandardAxis=+Z  RotationAngle=0  RotationArbitraryAxis=[0 0 1]  FollAlignAxisA=+X  BaseAlignAxisA=+Y  FollAlignAxisB=+Y  BaseAlignAxisB=+Z  RotationSequenceAxes=FollowerAxes  RotationSequence=XYX  RotationSequenceAngles=[0 0 0]  RotationSequenceAnglesUnits=deg  RotationMatrix=[1 0 0; 0 1 0; 0 0 1]
  Transform5 : sm_lib/Frames and Transforms/Rigid Transform  TranslationMethod=Cartesian  TranslationStandardOffset=0  TranslationLengthUnit=mm  TranslationStandardAxis=+Z  TranslationCartesianOffset=[-550 215 -60]  TranslationROffset=0  TranslationROffsetUnits=m  TranslationZOffset=0  TranslationZOffsetUnits=m  TranslationThetaOffset=0  TranslationThetaOffsetUnits=deg  RotationMethod=ArbitraryAxis  RotationAngleUnits=rad  RotationStandardAxis=+Z  RotationAngle=3.1415926535897896  RotationArbitraryAxis=[-1 -0 -1.99581e-15]  FollAlignAxisA=+X  BaseAlignAxisA=+Y  FollAlignAxisB=+Y  BaseAlignAxisB=+Z  RotationSequenceAxes=FollowerAxes  RotationSequence=XYX  RotationSequenceAngles=[0 0 0]  RotationSequenceAnglesUnits=deg  RotationMatrix=[1 0 0; 0 1 0; 0 0 1]
  Transform6 : sm_lib/Frames and Transforms/Rigid Transform  TranslationMethod=Cartesian  TranslationStandardOffset=0  TranslationLengthUnit=mm  TranslationStandardAxis=+Z  TranslationCartesianOffset=[20 -415 31]  TranslationROffset=0  TranslationROffsetUnits=m  TranslationZOffset=0  TranslationZOffsetUnits=m  TranslationThetaOffset=0  TranslationThetaOffsetUnits=deg  RotationMethod=ArbitraryAxis  RotationAngleUnits=rad  RotationStandardAxis=+Z  RotationAngle=3.1415926535897931  RotationArbitraryAxis=[0 -1.9146e-15 1]  FollAlignAxisA=+X  BaseAlignAxisA=+Y  FollAlignAxisB=+Y  BaseAlignAxisB=+Z  RotationSequenceAxes=FollowerAxes  RotationSequence=XYX  RotationSequenceAngles=[0 0 0]  RotationSequenceAnglesUnits=deg  RotationMatrix=[1 0 0; 0 1 0; 0 0 1]
  Transform7 : sm_lib/Frames and Transforms/Rigid Transform  TranslationMethod=Cartesian  TranslationStandardOffset=0  TranslationLengthUnit=mm  TranslationStandardAxis=+Z  TranslationCartesianOffset=[-1740 415 31]  TranslationROffset=0  TranslationROffsetUnits=m  TranslationZOffset=0  TranslationZOffsetUnits=m  TranslationThetaOffset=0  TranslationThetaOffsetUnits=deg  RotationMethod=None  RotationAngleUnits=deg  RotationStandardAxis=+Z  RotationAngle=0  RotationArbitraryAxis=[0 0 1]  FollAlignAxisA=+X  BaseAlignAxisA=+Y  FollAlignAxisB=+Y  BaseAlignAxisB=+Z  RotationSequenceAxes=FollowerAxes  RotationSequence=XYX  RotationSequenceAngles=[0 0 0]  RotationSequenceAnglesUnits=deg  RotationMatrix=[1 0 0; 0 1 0; 0 0 1]
  Transform8 : sm_lib/Frames and Transforms/Rigid Transform  TranslationMethod=Cartesian  TranslationStandardOffset=0  TranslationLengthUnit=mm  TranslationStandardAxis=+Z  TranslationCartesianOffset=[-760 275 -60]  TranslationROffset=0  TranslationROffsetUnits=m  TranslationZOffset=0  TranslationZOffsetUnits=m  TranslationThetaOffset=0  TranslationThetaOffsetUnits=deg  RotationMethod=ArbitraryAxis  RotationAngleUnits=rad  RotationStandardAxis=+Z  RotationAngle=1.5707963267948968  RotationArbitraryAxis=[-5.5510999999999988e-17 5.5510999999999988e-17 1]  FollAlignAxisA=+X  BaseAlignAxisA=+Y  FollAlignAxisB=+Y  BaseAlignAxisB=+Z  RotationSequenceAxes=FollowerAxes  RotationSequence=XYX  RotationSequenceAngles=[0 0 0]  RotationSequenceAnglesUnits=deg  RotationMatrix=[1 0 0; 0 1 0; 0 0 1]
  Transform9 : sm_lib/Frames and Transforms/Rigid Transform  TranslationMethod=Cartesian  TranslationStandardOffset=0  TranslationLengthUnit=mm  TranslationStandardAxis=+Z  TranslationCartesianOffset=[20 415 31]  TranslationROffset=0  TranslationROffsetUnits=m  TranslationZOffset=0  TranslationZOffsetUnits=m  TranslationThetaOffset=0  TranslationThetaOffsetUnits=deg  RotationMethod=ArbitraryAxis  RotationAngleUnits=rad  RotationStandardAxis=+Z  RotationAngle=3.1415926535897931  RotationArbitraryAxis=[0 -1.6751650000000001e-15 1]  FollAlignAxisA=+X  BaseAlignAxisA=+Y  FollAlignAxisB=+Y  BaseAlignAxisB=+Z  RotationSequenceAxes=FollowerAxes  RotationSequence=XYX  RotationSequenceAngles=[0 0 0]  RotationSequenceAnglesUnits=deg  RotationMatrix=[1 0 0; 0 1 0; 0 0 1]
  x15060_Coffret_elect_300_X_150_H_150_AA_DEFAULT_1_RIGID : Subsystem
  x15060_M_01006_Ens_pied_escamotable_Default_1_RIGID : Subsystem
  x15060_M_01006_Ens_pied_escamotable_Default_2_RIGID : Subsystem
  x15060_M_01006_Ens_pied_escamotable_Default_3_RIGID : Subsystem
  x15060_M_01006_Ens_pied_escamotable_Default_4_RIGID : Subsystem
  x15060_M_01009_Ens_chassis_inf_Default_1_RIGID : Subsystem
  x15060_M_01013_Ens_Coffret_electrique_sous_table_Default_1_RIGI : Subsystem
  x15060_M_01018_Ch_ssis_bas_1_RIGID : Subsystem
  x15060_M_01066_Protection_capteur_pied_AA_DEFAULT_1_RIGID : Subsystem
  x15060_M_01066_Protection_capteur_pied_AA_DEFAULT_2_RIGID : Subsystem
  x15060_M_01067_Protection_capteur_pied_SYM_AA_DEFAULT_1_RIGID : Subsystem
  x15060_M_01067_Protection_capteur_pied_SYM_AA_DEFAULT_2_RIGID : Subsystem
  x15060_M_01070_Plaquette_porte_coffret_elect_AA_DEFAULT_1_RIGID : Subsystem
  x15060_M_01070_Plaquette_porte_coffret_elect_AA_DEFAULT_2_RIGID : Subsystem
  x15060_M_01070_Plaquette_porte_coffret_elect_AA_DEFAULT_3_RIGID : Subsystem
  x15060_M_01070_Plaquette_porte_coffret_elect_AA_DEFAULT_4_RIGID : Subsystem
  F : PMIOPort  Side=Right
  F3 : PMIOPort  Port=2  Side=Left
  F2 : PMIOPort  Port=3  Side=Right
  F1 : PMIOPort  Port=4  Side=Right
  connections:
  Transform8/LConn1 -- Transform9/LConn1 -- Transform/LConn1 -- Transform1/LConn1 -- ReferenceFrame/RConn1 -- x15060_M_01013_Ens_Coffret_electrique_sous_table_Default_1_RIGI/RConn1 -- x15060_M_01018_Ch_ssis_bas_1_RIGID/RConn1 -- x15060_M_01009_Ens_chassis_inf_Default_1_RIGID/RConn1 -- x15060_M_01006_Ens_pied_escamotable_Default_4_RIGID/RConn1 -- x15060_M_01006_Ens_pied_escamotable_Default_3_RIGID/RConn1 -- x15060_M_01006_Ens_pied_escamotable_Default_2_RIGID/RConn1 -- x15060_M_01006_Ens_pied_escamotable_Default_1_RIGID/RConn1 -- F3/RConn1 -- Transform10/LConn1 -- Transform11/LConn1 -- Transform2/LConn1 -- Transform3/LConn1 -- Transform4/LConn1 -- Transform5/LConn1 -- Transform6/LConn1 -- Transform7/LConn1
  Transform/RConn1 -- F/RConn1
  Transform9/RConn1 -- x15060_M_01066_Protection_capteur_pied_AA_DEFAULT_2_RIGID/LConn1
  Transform10/RConn1 -- x15060_M_01070_Plaquette_porte_coffret_elect_AA_DEFAULT_4_RIGID/LConn1
  Transform11/RConn1 -- x15060_M_01070_Plaquette_porte_coffret_elect_AA_DEFAULT_3_RIGID/LConn1
  Transform1/RConn1 -- F1/RConn1
  Transform2/RConn1 -- F2/RConn1
  Transform3/RConn1 -- x15060_M_01070_Plaquette_porte_coffret_elect_AA_DEFAULT_2_RIGID/LConn1
  Transform4/RConn1 -- x15060_M_01066_Protection_capteur_pied_AA_DEFAULT_1_RIGID/LConn1
  Transform5/RConn1 -- x15060_M_01070_Plaquette_porte_coffret_elect_AA_DEFAULT_1_RIGID/LConn1
  Transform6/RConn1 -- x15060_M_01067_Protection_capteur_pied_SYM_AA_DEFAULT_1_RIGID/LConn1
  Transform7/RConn1 -- x15060_M_01067_Protection_capteur_pied_SYM_AA_DEFAULT_2_RIGID/LConn1
  Transform8/RConn1 -- x15060_Coffret_elect_300_X_150_H_150_AA_DEFAULT_1_RIGID/LConn1
